simulink model "modelcomparewithrobot"  (R2013a)
settings: Solver=ode4  StartTime=0.0  StopTime=10.0  FixedStep=0.005  RelTol=1e-3
libraries: simulink x1
settings Model: Creator=gkharish  LastModifiedBy=gkharish

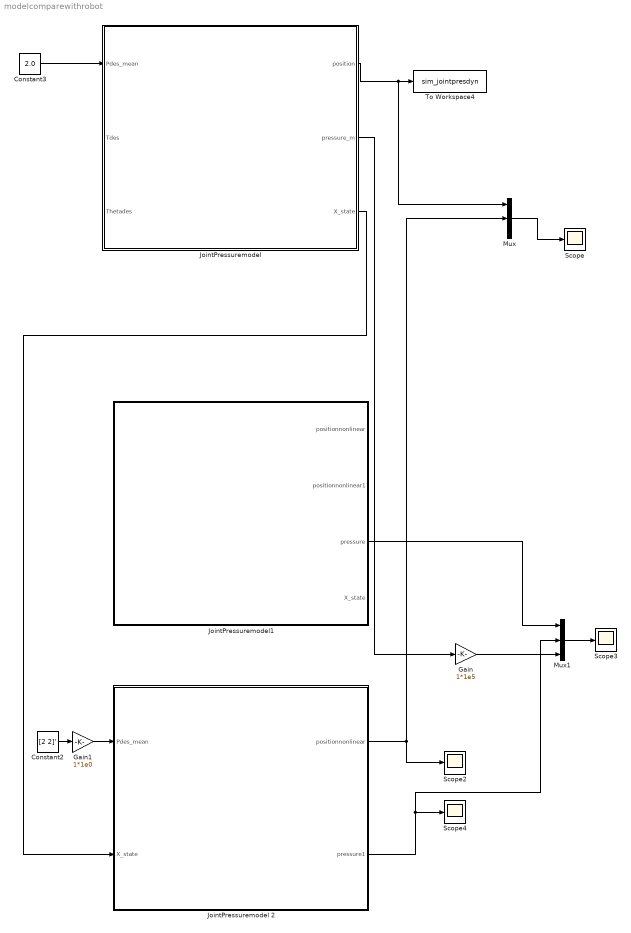
== system modelcomparewithrobot ==
  Constant2 : Constant  Value=[2 2]'
  Constant3 : Constant  Value=2.0
  Gain : Gain  Gain=1*1e5
  Gain1 : Gain  Gain=1*1e0
  "JointPressuremodel " : Subsystem
  JointPressuremodel 2 : Subsystem
  JointPressuremodel1 : Subsystem
  Mux : Mux  Inputs=3
  Mux1 : Mux  Inputs=3
  Scope{,2..4} (4 alike) : Scope
      Scope settings: ShowLegends=on  SaveName=ScopeData4
      Scope2 settings: SaveName=ScopeData10
      Scope3 settings: ShowLegends=on  SaveName=ScopeData15
      Scope4 settings: SaveName=ScopeData14
  To Workspace4 : ToWorkspace  VariableName=sim_jointpresdyn  SampleTime=-1  SaveFormat=Timeseries
  wires:
  Constant3/1 -> "JointPressuremodel "/1("Pdes_mean ")
  "JointPressuremodel "/1(position) -> Mux/1, To Workspace4/1
  Mux/1 -> Scope/1
  JointPressuremodel 2/1(positionnonlinear) -> Scope2/1, Mux/2
  JointPressuremodel 2/2(pressure1) -> Mux1/2, Scope4/1
  Mux1/1 -> Scope3/1
  "JointPressuremodel "/2(pressure_m) -> Gain/1
  JointPressuremodel1/3(pressure) -> Mux1/1
  Gain/1 -> Mux1/3
  Constant2/1 -> Gain1/1
  Gain1/1 -> JointPressuremodel 2/1("Pdes_mean ")
  "JointPressuremodel "/3(X_state) -> JointPressuremodel 2/2(X_state)

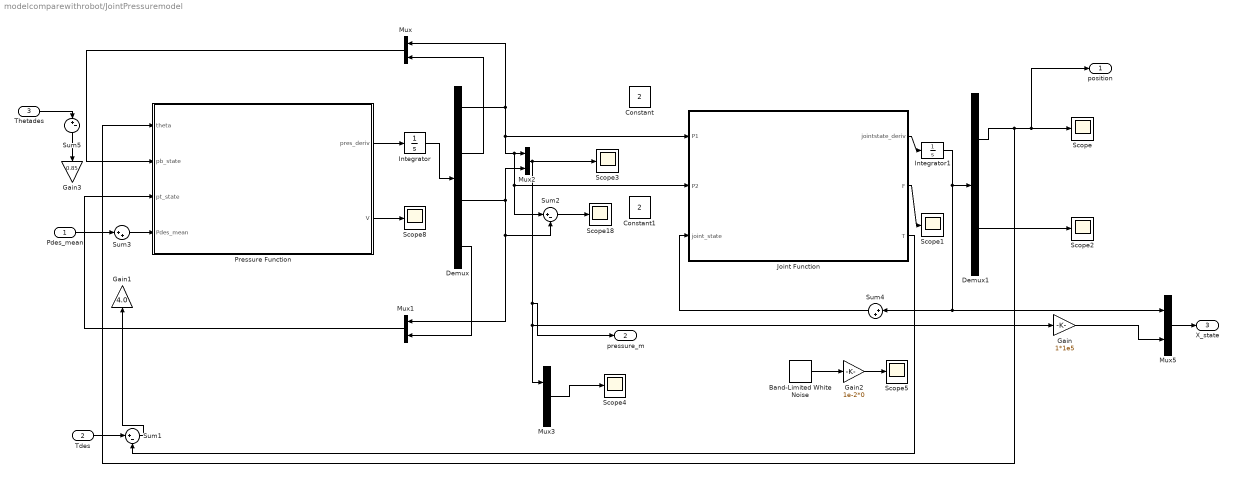
== system modelcomparewithrobot/JointPressuremodel  ==
  "Pdes_mean " : Inport
  Tdes : Inport  Port=2
  Thetades : Inport  Port=3
  Band-Limited White Noise : simulink/Sources/Band-Limited White Noise  Cov=[0.1]  Ts=0.005  seed=[23341]
  Constant : Constant  Value=2
  Constant1 : Constant  Value=2
  Demux : Demux
  Demux1 : Demux  Outputs=2
  Gain : Gain  Gain=1*1e5
  Gain1 : Gain  Gain=4.0
  Gain2 : Gain  Gain=1e-2*0
  Gain3 : Gain  Gain=0.85
  Integrator : Integrator  InitialCondition=[0 0 4 0]
  Integrator1 : Integrator  InitialCondition=[0 0]
  Joint Function : MATLAB Function  TreatAsAtomicUnit=on
  Mux{,1..3,5} (5 alike) : Mux  Inputs=2
  Pressure Function : MATLAB Function  TreatAsAtomicUnit=on
  Scope{,1..5,8,18} (8 alike) : Scope
      Scope settings: ShowLegends=on
      Scope1 settings: ShowLegends=on  TimeRange=10  YMin=240  YMax=285
      Scope18 settings: ShowLegends=on  SaveName=ScopeData18
      Scope2 settings: SaveName=ScopeData2
      Scope3 settings: ShowLegends=on  SaveName=ScopeData3
      Scope4 settings: ShowLegends=on  SaveName=ScopeData25
      Scope5 settings: ShowLegends=on  SaveName=ScopeData27
      Scope8 settings: ShowLegends=on  SaveName=ScopeData8
  Sum1 : Sum  Inputs=|+-
  Sum2 : Sum  Inputs=|+-
  Sum3 : Sum  Inputs=|++
  Sum4 : Sum  Inputs=|++
  Sum5 : Sum  Inputs=|+-
  position : Outport
  pressure_m : Outport  Port=2
  X_state : Outport  Port=3
  wires:
  Demux/1 -> Joint Function/1(P1), Joint Function/2(P2), Sum2/1, Mux2/1, Mux/1
  Integrator1/1 -> Mux5/1, Sum4/1, Demux1/1
  Pressure Function/2(V) -> Scope8/1
  Mux1/1 -> Pressure Function/3(pt_state)
  Demux/2 -> Mux/2
  Joint Function/1(jointstate_deriv) -> Integrator1/1
  Demux/4 -> Mux1/2
  Demux1/2 -> Scope2/1
  Demux1/1 -> Pressure Function/1(theta), position/1, Scope/1
  Joint Function/2(F) -> Scope1/1
  Pressure Function/1(pres_deriv) -> Integrator/1
  Mux/1 -> Pressure Function/2(pb_state)
  Integrator/1 -> Demux/1
  Sum2/1 -> Scope18/1
  Demux/3 -> Sum2/2, Mux1/1, Mux2/2
  Mux3/1 -> Scope4/1
  "Pdes_mean "/1 -> Sum3/1
  Sum3/1 -> Pressure Function/4(Pdes_mean)
  Sum1/1 -> Gain1/1
  Mux2/1 -> Scope3/1, pressure_m/1, Mux3/1, Gain/1
  Joint Function/3(T) -> Sum1/2
  Band-Limited White Noise/1 -> Gain2/1
  Sum4/1 -> Joint Function/3(joint_state)
  Gain2/1 -> Scope5/1
  Tdes/1 -> Sum1/1
  Thetades/1 -> Sum5/1
  Sum5/1 -> Gain3/1
  Mux5/1 -> X_state/1
  Gain/1 -> Mux5/2

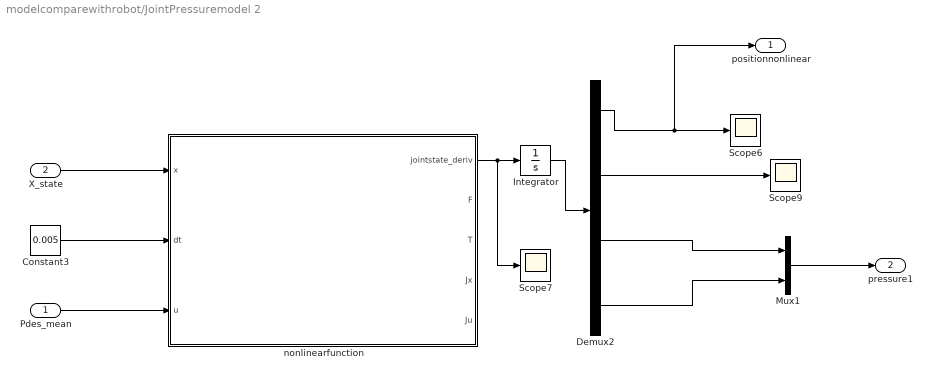
== system modelcomparewithrobot/JointPressuremodel 2 ==
  "Pdes_mean " : Inport
  X_state : Inport  Port=2
  Constant3 : Constant  Value=0.005
  Demux2 : Demux
  Integrator : Integrator  InitialCondition=[0 0 0 4]
  Mux1 : Mux  Inputs=2
  Scope6 : Scope
      settings: ShowLegends=on  SaveName=ScopeData5
  Scope7 : Scope
      settings: ShowLegends=on  TimeRange=10  YMin=240  YMax=285  SaveName=ScopeData6
  Scope9 : Scope
      settings: SaveName=ScopeData7
  "nonlinearfunction " : MATLAB Function  TreatAsAtomicUnit=on
  positionnonlinear : Outport
  pressure1 : Outport  Port=2
  wires:
  Demux2/2 -> Scope9/1
  Demux2/1 -> Scope6/1, positionnonlinear/1
  "Pdes_mean "/1 -> "nonlinearfunction "/3(u)
  Constant3/1 -> "nonlinearfunction "/2(dt)
  "nonlinearfunction "/1(jointstate_deriv) -> Scope7/1, Integrator/1
  Demux2/4 -> Mux1/2
  Demux2/3 -> Mux1/1
  Mux1/1 -> pressure1/1
  Integrator/1 -> Demux2/1
  X_state/1 -> "nonlinearfunction "/1(x)

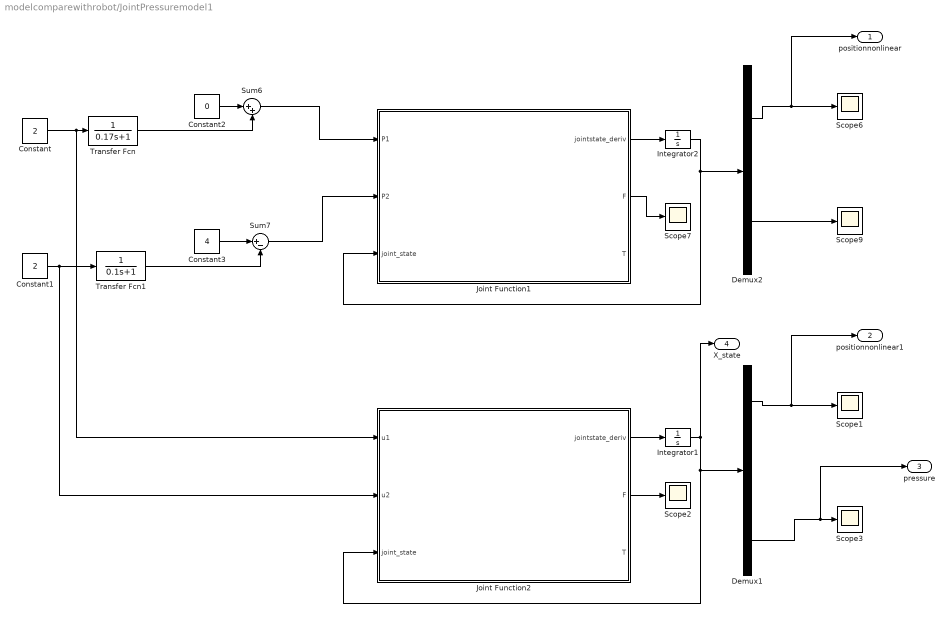
== system modelcomparewithrobot/JointPressuremodel1 ==
  Constant : Constant  Value=2
  Constant1 : Constant  Value=2
  Constant2 : Constant  Value=0
  Constant3 : Constant  Value=4
  Demux1 : Demux  Outputs=[1 1 2]
  Demux2 : Demux  Outputs=2
  Integrator1 : Integrator  InitialCondition=[0 0 0 4*1e5]
  Integrator2 : Integrator  InitialCondition=[0 0]
  Joint Function1 : MATLAB Function  TreatAsAtomicUnit=on
  Joint Function2 : MATLAB Function  TreatAsAtomicUnit=on
  Scope{1..3,6..7,9} (6 alike) : Scope
      Scope1 settings: ShowLegends=on  SaveName=ScopeData11
      Scope2 settings: ShowLegends=on  TimeRange=10  YMin=240  YMax=285  SaveName=ScopeData12
      Scope3 settings: SaveName=ScopeData13
      Scope6 settings: ShowLegends=on  SaveName=ScopeData5
      Scope7 settings: ShowLegends=on  TimeRange=10  YMin=240  YMax=285  SaveName=ScopeData6
      Scope9 settings: SaveName=ScopeData7
  Sum6 : Sum  Inputs=|++
  Sum7 : Sum  Inputs=|+-
  Transfer Fcn : TransferFcn  Denominator=[0.17 1]
  Transfer Fcn1 : TransferFcn  Denominator=[0.1 1]
  positionnonlinear : Outport
  positionnonlinear1 : Outport  Port=2
  pressure : Outport  Port=3
  X_state : Outport  Port=4
  wires:
  Demux2/1 -> positionnonlinear/1, Scope6/1
  Demux2/2 -> Scope9/1
  Integrator2/1 -> Joint Function1/3(joint_state), Demux2/1
  Joint Function1/1(jointstate_deriv) -> Integrator2/1
  Joint Function1/2(F) -> Scope7/1
  Transfer Fcn/1 -> Sum6/2
  Constant2/1 -> Sum6/1
  Sum6/1 -> Joint Function1/1(P1)
  Transfer Fcn1/1 -> Sum7/2
  Constant3/1 -> Sum7/1
  Sum7/1 -> Joint Function1/2(P2)
  Constant1/1 -> Joint Function2/2(u2), Transfer Fcn1/1
  Constant/1 -> Joint Function2/1(u1), Transfer Fcn/1
  Demux1/1 -> Scope1/1, positionnonlinear1/1
  Integrator1/1 -> Demux1/1, Joint Function2/3(joint_state), X_state/1
  Joint Function2/1(jointstate_deriv) -> Integrator1/1
  Joint Function2/2(F) -> Scope2/1
  Demux1/3 -> pressure/1, Scope3/1

== matlab function modelcomparewithrobot/JointPressuremodel /Joint Function ==
  data: P1 input; jointstate_deriv output; P2 input; joint_state input; F output; T output
function [jointstate_deriv,F, T] = jointdynamics(P1, P2, joint_state)
jointstate_deriv = zeros(2,1);
theta = joint_state(1);
theta_dot = joint_state(2);
%% Parameters for the muscles
lo = 0.185;
alphao = 23.0*pi/180;
%epsilono = 0.15;
%emax = 0.2983;
k = 1.25;
ro = 0.0085;
R = 0.015;

a = 3/(tan(alphao))^2;
b = 1/(sin(alphao))^2;
emax = (1/k)*(1 - sqrt(b/a));

lb = lo- R*theta;
epsb = (1-(lb/lo));
lt = lo*(1-emax) + R*theta;
epst = (1-(lt/lo));

%% Parameters of Joint
m = 2.6;
link_l = 0.32;
g =9.81;
I = m*(link_l^2)/3;
fv = 0.25;


F1 =  pi*ro^2*P1*1e5*(a*(1-k*epsb)^2 - b);
F2 =  pi*ro^2*P2*1e5*(a*(1-k*epst)^2 - b);
F2max = 1*pi*ro^2*4*1e5*(a*(1-k*emax)^2 - b);
T = (F1 -F2 )*R;
F = [F1 F2 T];
jointstate_deriv(1) = theta_dot; %joint_state(2);
jointstate_deriv(2) = ((F1 -F2 )*R  - fv*theta_dot - m*g*0.5*link_l*sin(theta))/I;

== matlab function modelcomparewithrobot/JointPressuremodel /Pressure Function ==
  data: theta input; pres_deriv output; pb_state input; pt_state input; Pdes_mean input; V output
function [pres_deriv,V] = pressuredynamics(theta, pb_state, pt_state, Pdes_mean)

pres_deriv = zeros(4,1);
V = zeros(2,1);
Pdes = zeros(2,1);
%% Parameters for the muscles
lo = 0.185;
alphao = 23.0*pi/180;
%epsilono = 0.15;
%emax = 0.2983;
k = 1.25;
ro = 0.0085;
R = 0.015;
a = 3/(tan(alphao))^2;
b = 1/(sin(alphao))^2;
emax = (1/k)*(1 - sqrt(b/a));
%% Calculate Volume 
% biceps agonistic muscle
lb = lo - R*theta;
cs2 = (cos(alphao))^2;
epsb2 = (1-(lb/lo))^2;
termb1 = (1 - cs2*epsb2);

Vb = 1e6*(pi*lb*ro^2/((sin(alphao))^2))*termb1;
%Vb = 230;
wnb = 2*pi*380*(1/Vb);

% triceps antagonistic muscle 
lt = lo*(1-emax) + R*theta; 
cs2 = (cos(alphao))^2;
epst2 = (1-(lt/lo))^2;
termt1 = (1 - cs2*epst2);

Vt = 1e6*(pi*lt*ro^2/((sin(alphao))^2))*termt1;
%Vt = 230;
wnt = 2*pi*380*(1/Vt);

Pdes(1) = Pdes_mean;
Pdes(2) = 4 - Pdes_mean;

pres_deriv(1) = pb_state(2);
pres_deriv(2) = -wnb^2*pb_state(1) - 2*wnb*1*pb_state(2) + (wnb^2)*Pdes(1);

pres_deriv(3) = pt_state(2);
pres_deriv(4) = -wnt^2*pt_state(1) - 2*wnt*1*pt_state(2) + (wnt^2)*Pdes(2);

% pres_deriv(5) = Vb;
% pres_deriv(6) = Vt;
V = [wnb;wnt];

== matlab function modelcomparewithrobot/JointPressuremodel1/Joint Function2 ==
  data: u1 input; jointstate_deriv output; u2 input; joint_state input; F output; T output
function [jointstate_deriv,F, T] = jointdynamics(u1,u2,joint_state)
jointstate_deriv = zeros(4,1);
theta = joint_state(1);
theta_dot = joint_state(2);
P1 = joint_state(3);
P2 = joint_state(4);
%% Parameters for the muscles
lo = 0.185;
alphao = 23.0*pi/180;
%epsilono = 0.15;
%emax = 0.2983;
k = 1.25;
ro = 0.0085;
R = 0.015;

a = 3/(tan(alphao))^2;
b = 1/(sin(alphao))^2;
emax = (1/k)*(1 - sqrt(b/a));

lb = lo- R*theta;
epsb = (1-(lb/lo));
lt = lo*(1-emax) + R*theta;
epst = (1-(lt/lo));

%% Parameters of Joint
m = 2.6;
link_l = 0.32;
g =9.81;
I = m*(link_l^2)/3;
fv = 0.25;


F1 =  pi*ro^2*P1*(a*(1-k*epsb)^2 - b);
F2 =  pi*ro^2*P2*(a*(1-k*epst)^2 - b);
F2max = 1*pi*ro^2*4*1e5*(a*(1-k*emax)^2 - b);
T = (F1 -F2 )*R;
F = [F1 F2 T];


%% Non linear modelling
Tc2 =0.13; 
Tc1 = 0.19;
% co = pi*ro^2;
% tb1 = co*(a -b)*P1;
% tb2 = co*a*(-2*k)*(R/lo)*P1*theta;
% tb3 = co*a*(k^2*R^2/(lo^2))*P1*(theta^2);
% F1 = tb1 + tb2 + tb3;
% 
% tt1 = co*(a -b)*P2;
% 
% tt2_1 = (k*emax)^2 - 2*k*emax;
% tt2 = co*a*tt2_1*P2;
% 
% tt3_1 = (R*theta/lo)^2 - 2*emax*(R*theta/lo);
% 
% tt3 = co*a*(k^2*tt3_1 + 2*k*(R*theta/lo))*P2;
% 
% F2 = tt1 +tt2 +tt3;
% 
% T = (F1 -F2 )*R;
% F = [F1 F2 T];

jointstate_deriv(1) = theta_dot; %joint_state(2);
jointstate_deriv(2) = ((F1 -F2 )*R  - fv*theta_dot - m*g*0.5*link_l*sin(theta))/I;
jointstate_deriv(3) = -P1/Tc1 + u1*1e5/Tc1;
jointstate_deriv(4) = -P2/Tc2 + u2*1e5/Tc2;

== matlab function modelcomparewithrobot/JointPressuremodel1/Joint Function1 ==
  data: P1 input; jointstate_deriv output; P2 input; joint_state input; F output; T output
function [jointstate_deriv,F, T] = jointdynamics(P1, P2, joint_state)
jointstate_deriv = zeros(2,1);
theta = joint_state(1);
theta_dot = joint_state(2);
%% Parameters for the muscles
lo = 0.185;
alphao = 23.0*pi/180;
%epsilono = 0.15;
%emax = 0.2983;
k = 1.25;
ro = 0.0085;
R = 0.015;

a = 3/(tan(alphao))^2;
b = 1/(sin(alphao))^2;
emax = (1/k)*(1 - sqrt(b/a));

lb = lo- R*theta;
epsb = (1-(lb/lo));
lt = lo*(1-emax) + R*theta;
epst = (1-(lt/lo));

%% Parameters of Joint
m = 2.6;
link_l = 0.32;
g =9.81;
I = m*(link_l^2)/3;
fv = 0.25;


% F1 =  pi*ro^2*P1*1e5*(a*(1-k*epsb)^2 - b);
% F2 =  pi*ro^2*P2*1e5*(a*(1-k*epst)^2 - b);
% F2max = 1*pi*ro^2*4*1e5*(a*(1-k*emax)^2 - b);
% T = (F1 -F2 )*R;
% F = [F1 F2 T];


%% Non linear modelling

co = pi*ro^2*1e5;
tb1 = co*(a -b)*P1;
tb2 = co*a*(-2*k)*(R/lo)*P1*theta;
tb3 = co*a*(k^2*R^2/(lo^2))*P1*(theta^2);
F1 = tb1 + tb2 + tb3;

tt1 = co*(a -b)*P2;

tt2_1 = (k*emax)^2 - 2*k*emax;
tt2 = co*a*tt2_1*P2;

tt3_1 = (R*theta/lo)^2 - 2*emax*(R*theta/lo);

tt3 = co*a*(k^2*tt3_1 + 2*k*(R*theta/lo))*P2;

F2 = tt1 +tt2 +tt3;

T = (F1 -F2 )*R;
F = [F1 F2 T];

jointstate_deriv(1) = theta_dot; %joint_state(2);
jointstate_deriv(2) = ((F1 -F2 )*R  - fv*theta_dot - m*g*0.5*link_l*sin(theta))/I;

== matlab function modelcomparewithrobot/JointPressuremodel 2/nonlinearfunction  ==
  data: jointstate_deriv output; x input; F output; T output; Jx output; Ju output; dt input; u input
function [jointstate_deriv,F, T, Jx, Ju] = jointdynamics(x, dt,u)
jointstate_deriv = zeros(4,1);
joint_state = zeros(4,1);
joint_state =x;
theta = joint_state(1);
theta_dot = joint_state(2);
P1 = joint_state(3);
P2 = joint_state(4);
%% Parameters for the muscles
lo = 0.185;
alphao = 23.0*pi/180;
%epsilono = 0.15;
%emax = 0.2983;
k = 1.25;
ro = 0.0085;
R = 0.015;

a = 3/(tan(alphao))^2;
b = 1/(sin(alphao))^2;
emax = (1/k)*(1 - sqrt(b/a));

lb = lo- R*theta;
epsb = (1-(lb/lo));
lt = lo*(1-emax) + R*theta;
epst = (1-(lt/lo));

%% Parameters of Joint
m = 2.6;
link_l = 0.32;
g =9.81;
I = m*(link_l^2)/3;
fv = 0.25;


% F1 =  pi*ro^2*P1*1e5*(a*(1-k*epsb)^2 - b);
% F2 =  pi*ro^2*P2*1e5*(a*(1-k*epst)^2 - b);
% F2max = 1*pi*ro^2*4*1e5*(a*(1-k*emax)^2 - b);
% T = (F1 -F2 )*R;
% F = [F1 F2 T];


%% Non linear modelling

co = pi*ro^2;
tb1 = co*(a -b)*P1;
tb2 = co*a*(-2*k)*(R/lo)*P1*theta;
tb3 = co*a*(k^2*R^2/(lo^2))*P1*(theta^2);
F1 = tb1 + tb2 + tb3;

tt1 = co*(a -b)*P2;

tt2_1 = (k*emax)^2 - 2*k*emax;
tt2 = co*a*tt2_1*P2;

tt3_1 = (R*theta/lo)^2 - 2*emax*(R*theta/lo);

tt3 = co*a*(k^2*tt3_1 + 2*k*(R*theta/lo))*P2;

F2 = tt1 +tt2 +tt3;

T = (F1 -F2 )*R;
F = [F1 F2 T];

% jointstate_deriv(1) = theta_dot; %joint_state(2);
% jointstate_deriv(2) = ((F1 -F2 )*R  - fv*theta_dot - m*g*0.5*link_l*sin(theta))/I;

%% Calculation of Jacobian
% Tc1 = 0.18;
% Tc2 = 0.13;
% Jx = zeros(4,4);
% Jx(1,:) = [0 1 0 0];
% Jx(3,:) = [0 0 (-1/Tc1) 0];
% Jx(4,:) = [0 0 0 (-1/Tc2)];

% %% J(2,1)
% 
% t1_j21  = - m*g*0.5*link_l*cos(theta)/I;
% t2_j21 = 2*co*a*k^2*emax*(R/lo)*P2;
% t3_j21 = 2*co*a*((k*R/lo)^2)*(P1 - P2)*theta;
% t4_j21 = -2*co*a*k*(R/lo)*(P1 + P2);
% Jx(2,1) = t1_j21 + (t2_j21 + t3_j21 + t4_j21)*(R/I);
% %% J(2,2)
% Jx(2,2) = -fv/I;
% %% J(2,3)
% 
% t1_j23 = co*(a-b);
% t2_j23 = -2*co*a*k*(R/lo)*theta;
% t3_j23 = co*a*((k*R/lo)^2)*theta^2;
% 
% Jx(2,3) = (t1_j23  + t2_j23 + t3_j23 )*(R/I);
% %% j(2,4)
% 
% t1_j24 =co*(a-b);
% 
% t2_j24 = co*a*((k*emax)^2 - 2*k*emax);
% tt3_1 = (R*theta/lo)^2 - 2*emax*(R*theta/lo);
% 
% t3_j24 = co*a*(k^2*tt3_1 + 2*k*(R*theta/lo));
% 
% Jx(2,4) = -(t1_j24 + t2_j24 + t3_j24)*(R/I);

%% Alternative calculation of jacobian
Tc1 = 0.19;
Tc2 = 0.13;
Jx = zeros(4,4);
Jx(1,:) = [0 1 0 0];
Jx(3,:) = [0 0 (-1/Tc1) 0];
Jx(4,:) = [0 0 0 (-1/Tc2)];
t1_j21  = - m*g*0.5*link_l*cos(theta)/I;
 t1 = -pi*ro^2*P1*1e5*(2*a*k*(1-k*epsb)*(R/lo));
 t2 = -pi*ro^2*P2*1e5*(2*a*k*(1-k*epst)*(R/lo));
 Jx(2,1) = t1_j21 + (t1 + t2)*(R/I);
 Jx(2,2) = -fv/I;
 Jx(2,3) = (R/I)*pi*ro^2*(a*(1-k*epsb)^2 - b)*1e5;
 Jx(2,4) = (-R/I)*pi*ro^2*(a*(1-k*epst)^2 - b)*1e5;
% F2 =  pi*ro^2*P2*1e5*(a*(1-k*epst)^2 - b);

%%
Ju = zeros(4,2);
Ju(:,1) = [0 0 1/Tc1 0]';
Ju(:,2) = [0 0 0 1/Tc2]';
Ad = Jx*dt + eye(4);
Bd = Ju*dt;

Jx
jointstate_deriv = Jx*joint_state + Ju*u;
end
